simulink model "verificationsteeringplant"  (Simulink 7.9)
settings: Solver=ode45  StartTime=0.0  StopTime=10.0  RelTol=1e-3
undefined symbols (not defined in the file): Ks, offset
settings Model: Creator=rdestr15  LastModifiedBy=rdestr15

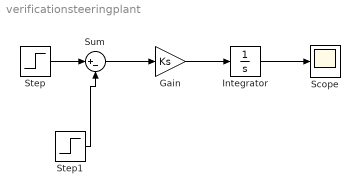
== system verificationsteeringplant ==
  Gain : Gain  Gain=Ks
  Integrator : Integrator
  Scope : Scope
  Step : Step  Time=5  Before=1360  After=1670  SampleTime=0
  Step1 : Step  Time=5  Before=1360  After=offset  SampleTime=0
  Sum : Sum  Inputs=|+-
  wires:
  Step/1 -> Sum/1
  Sum/1 -> Gain/1
  Gain/1 -> Integrator/1
  Integrator/1 -> Scope/1
  Step1/1 -> Sum/2
